simulink model "Md57TrgtPosChk"  (R2018b)
settings: Solver=FixedStepDiscrete  StartTime=0.0  StopTime=10.0  RelTol=1e-3
undefined symbols (not defined in the file or in its folder): Md57TrgtPos_Set, SecRwLtStBkReclnTrgtPos, SecRwLtStFwdBkwdTrgtPos, SecRwLtStLgrstInwdOtwdTrgtPos, SecRwLtStLgrstUpwdDnwdTrgtPos, SecRwLtStZeroTrgtPos
settings Model: Creator=sn2xws  LastModifiedBy=sn2xws
settings Model: ModifiedHistory=|
  | 2024.10.15 V3.0.0 Md57目标位置计算
  | 2024.11.27 V3.0.1 6s版本不看三左前后位置,无解时，使用最小智享位置
settings DataIOCC: SaveFormat=StructureWithTime
settings OptimizationCC: DefaultParameterBehavior=Inlined  EnhancedBackFolding=on  PassReuseOutputArgsAs=Individual arguments  ZeroExternalMemoryAtStartup=off  ZeroInternalMemoryAtStartup=off  OptimizeBlockOrder=speed  DifferentSizesBufferReuse=on  OptimizationCustomize=off
settings DebuggingCC: ParameterTunabilityLossMsg=error
settings SFSimCC: MATLABDynamicMemAlloc=off
settings SFSimCC: SimCustomHeaderCode=|
  | #include "qmath.h"
  | #include "MsminterfDet.h"
  | #include "wisenjoy.h"
settings SFSimCC: SimUserSources=|
  | qmath.c
  | MsminterfDet.c
  | wisenjoy.c
settings RTWCC: SystemTargetFile=autosar.tlc  GenCodeOnly=on  TemplateMakefile=ert_default_tmf  Description=AUTOSAR  GenerateReport=on  IncludeHyperlinkInReport=on  LaunchReport=on  GenerateTraceInfo=on  GenerateTraceReport=on  GenerateTraceReportSl=on  GenerateTraceReportSf=on  GenerateTraceReportEml=on
settings CodeAppCC: ForceParamTrailComments=on  IgnoreCustomStorageClasses=off  OperatorAnnotations=on  SimulinkDataObjDesc=on  SFDataObjDesc=on  InsertBlockDesc=on
settings STFCustomTargetCC: TargetLangStandard=C99 (ISO)  MultiwordLength=256  ParMdlRefBuildCompliant=on  CompOptLevelCompliant=on  IncludeMdlTerminateFcn=off  CombineOutputUpdateFcns=on  SuppressErrorStatus=on  ERTCustomFileBanners=on  SupportNonFinite=off  SupportComplex=off  SupportContinuousTime=off  SupportNonInlinedSFcns=off  RemoveResetFunc=on  MATLABClassNameForMDSCustomization=Simulink.SoftwareTarget.ERTCustomization  AutosarCompliant=on  UseToolchainInfoCompliant=on  LookupTableObjectStructAxisOrder=2,1,3,4,...  LUTObjectStructOrderEvenSpacing=Size,Table,Breakpoints  SystemTargetFile=autosar.tlc
settings ERTTargetCC: TargetLangStandard=C99 (ISO)  ConcurrentExecutionCompliant=off  IncludeMdlTerminateFcn=off  SuppressErrorStatus=on  SupportNonFinite=off  SupportComplex=off  ModelStepFunctionPrototypeControlCompliant=off  CPPClassGenCompliant=off  AutosarCompliant=on  LookupTableObjectStructAxisOrder=2,1,3,4,...  LUTObjectStructOrderEvenSpacing=Size,Table,Breakpoints  InlinedParameterPlacement=NonHierarchical  ERTCustomFileTemplate=example_file_process.tlc  ERTFilePackagingFormat=Compact

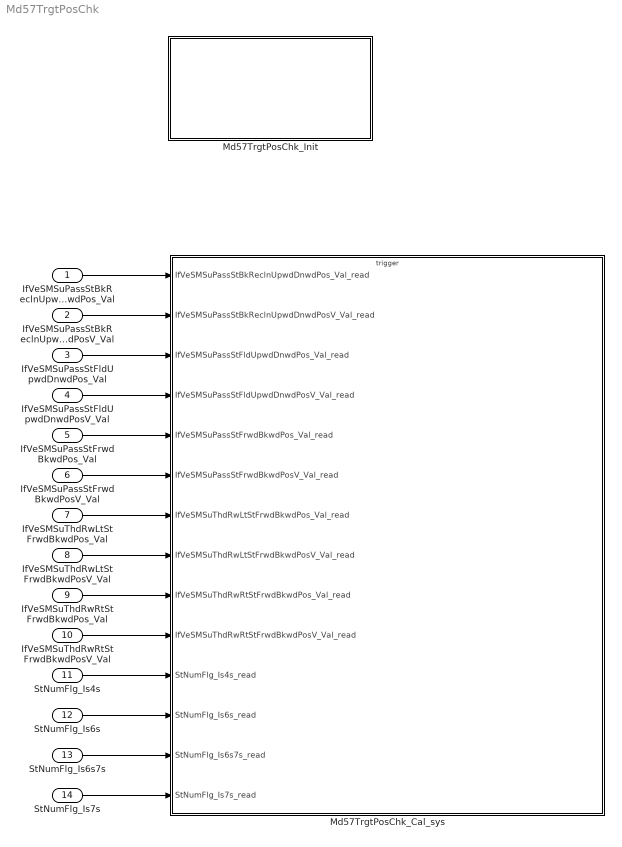
== system Md57TrgtPosChk ==
  IfVeSMSuPassStBkReclnUpwdDnwdPos_Val : Inport  OutDataTypeStr=uint16  PortDimensions=1
  IfVeSMSuPassStBkReclnUpwdDnwdPosV_Val : Inport  Port=2  OutDataTypeStr=boolean  PortDimensions=1
  IfVeSMSuPassStFldUpwdDnwdPos_Val : Inport  Port=3  OutDataTypeStr=uint16  PortDimensions=1
  IfVeSMSuPassStFldUpwdDnwdPosV_Val : Inport  Port=4  OutDataTypeStr=boolean  PortDimensions=1
  IfVeSMSuPassStFrwdBkwdPos_Val : Inport  Port=5  OutDataTypeStr=uint16  PortDimensions=1
  IfVeSMSuPassStFrwdBkwdPosV_Val : Inport  Port=6  OutDataTypeStr=boolean  PortDimensions=1
  IfVeSMSuThdRwLtStFrwdBkwdPos_Val : Inport  Port=7  OutDataTypeStr=uint16  PortDimensions=1
  IfVeSMSuThdRwLtStFrwdBkwdPosV_Val : Inport  Port=8  OutDataTypeStr=boolean  PortDimensions=1
  IfVeSMSuThdRwRtStFrwdBkwdPos_Val : Inport  Port=9  OutDataTypeStr=uint16  PortDimensions=1
  IfVeSMSuThdRwRtStFrwdBkwdPosV_Val : Inport  Port=10  OutDataTypeStr=boolean  PortDimensions=1
  StNumFlg_Is4s : Inport  Port=11  OutDataTypeStr=boolean  PortDimensions=1
  StNumFlg_Is6s : Inport  Port=12  OutDataTypeStr=boolean  PortDimensions=1
  StNumFlg_Is6s7s : Inport  Port=13  OutDataTypeStr=boolean  PortDimensions=1
  StNumFlg_Is7s : Inport  Port=14  OutDataTypeStr=boolean  PortDimensions=1
  Md57TrgtPosChk_Cal_sys : Subsystem
  Md57TrgtPosChk_Init : Subsystem
  wires:
  IfVeSMSuPassStBkReclnUpwdDnwdPos_Val/1 -> Md57TrgtPosChk_Cal_sys/1(IfVeSMSuPassStBkReclnUpwdDnwdPos_Val_read)
  IfVeSMSuPassStBkReclnUpwdDnwdPosV_Val/1 -> Md57TrgtPosChk_Cal_sys/2(IfVeSMSuPassStBkReclnUpwdDnwdPosV_Val_read)
  IfVeSMSuPassStFldUpwdDnwdPos_Val/1 -> Md57TrgtPosChk_Cal_sys/3(IfVeSMSuPassStFldUpwdDnwdPos_Val_read)
  IfVeSMSuPassStFldUpwdDnwdPosV_Val/1 -> Md57TrgtPosChk_Cal_sys/4(IfVeSMSuPassStFldUpwdDnwdPosV_Val_read)
  IfVeSMSuPassStFrwdBkwdPos_Val/1 -> Md57TrgtPosChk_Cal_sys/5(IfVeSMSuPassStFrwdBkwdPos_Val_read)
  IfVeSMSuPassStFrwdBkwdPosV_Val/1 -> Md57TrgtPosChk_Cal_sys/6(IfVeSMSuPassStFrwdBkwdPosV_Val_read)
  IfVeSMSuThdRwLtStFrwdBkwdPos_Val/1 -> Md57TrgtPosChk_Cal_sys/7(IfVeSMSuThdRwLtStFrwdBkwdPos_Val_read)
  IfVeSMSuThdRwLtStFrwdBkwdPosV_Val/1 -> Md57TrgtPosChk_Cal_sys/8(IfVeSMSuThdRwLtStFrwdBkwdPosV_Val_read)
  IfVeSMSuThdRwRtStFrwdBkwdPos_Val/1 -> Md57TrgtPosChk_Cal_sys/9(IfVeSMSuThdRwRtStFrwdBkwdPos_Val_read)
  IfVeSMSuThdRwRtStFrwdBkwdPosV_Val/1 -> Md57TrgtPosChk_Cal_sys/10(IfVeSMSuThdRwRtStFrwdBkwdPosV_Val_read)
  StNumFlg_Is4s/1 -> Md57TrgtPosChk_Cal_sys/11(StNumFlg_Is4s_read)
  StNumFlg_Is6s/1 -> Md57TrgtPosChk_Cal_sys/12(StNumFlg_Is6s_read)
  StNumFlg_Is6s7s/1 -> Md57TrgtPosChk_Cal_sys/13(StNumFlg_Is6s7s_read)
  StNumFlg_Is7s/1 -> Md57TrgtPosChk_Cal_sys/14(StNumFlg_Is7s_read)

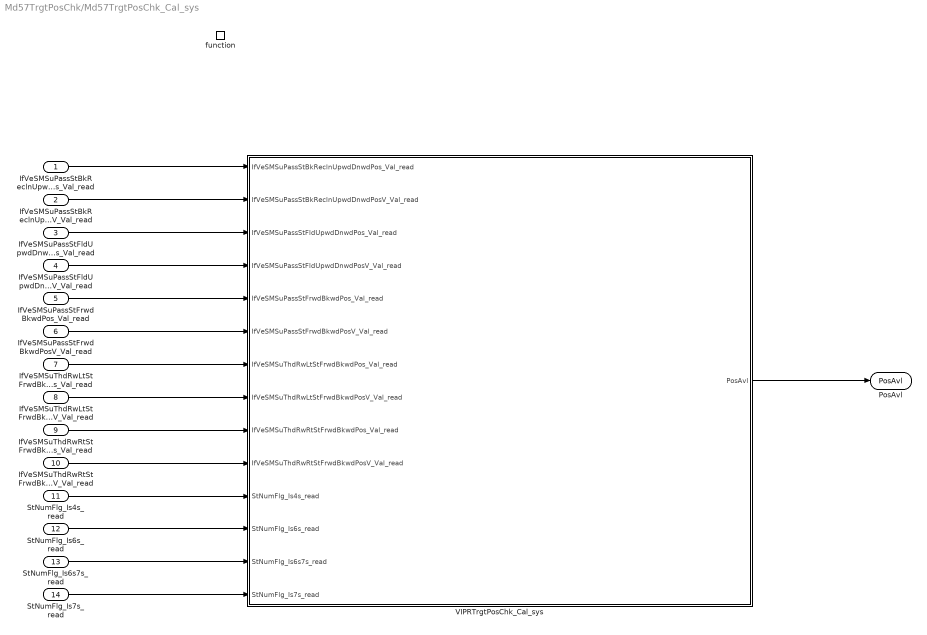
== system Md57TrgtPosChk/Md57TrgtPosChk_Cal_sys ==
  IfVeSMSuPassStBkReclnUpwdDnwdPos_Val_read : Inport
  IfVeSMSuPassStBkReclnUpwdDnwdPosV_Val_read : Inport  Port=2
  IfVeSMSuPassStFldUpwdDnwdPos_Val_read : Inport  Port=3
  IfVeSMSuPassStFldUpwdDnwdPosV_Val_read : Inport  Port=4
  IfVeSMSuPassStFrwdBkwdPos_Val_read : Inport  Port=5
  IfVeSMSuPassStFrwdBkwdPosV_Val_read : Inport  Port=6
  IfVeSMSuThdRwLtStFrwdBkwdPos_Val_read : Inport  Port=7
  IfVeSMSuThdRwLtStFrwdBkwdPosV_Val_read : Inport  Port=8
  IfVeSMSuThdRwRtStFrwdBkwdPos_Val_read : Inport  Port=9
  IfVeSMSuThdRwRtStFrwdBkwdPosV_Val_read : Inport  Port=10
  StNumFlg_Is4s_read : Inport  Port=11
  StNumFlg_Is6s_read : Inport  Port=12
  StNumFlg_Is6s7s_read : Inport  Port=13
  StNumFlg_Is7s_read : Inport  Port=14
  function : TriggerPort  TriggerType=function-call  IsSimulinkFunction=on  FunctionName=Md57TrgtPosChk_Cal  VariantControl=(inherit)
  VIPRTrgtPosChk_Cal_sys : Subsystem
  PosAvl : ArgOut  OutDataTypeStr=uint8  ArgumentName=PosAvl
  wires:
  IfVeSMSuPassStBkReclnUpwdDnwdPos_Val_read/1 -> VIPRTrgtPosChk_Cal_sys/1(IfVeSMSuPassStBkReclnUpwdDnwdPos_Val_read)
  IfVeSMSuPassStBkReclnUpwdDnwdPosV_Val_read/1 -> VIPRTrgtPosChk_Cal_sys/2(IfVeSMSuPassStBkReclnUpwdDnwdPosV_Val_read)
  IfVeSMSuPassStFldUpwdDnwdPos_Val_read/1 -> VIPRTrgtPosChk_Cal_sys/3(IfVeSMSuPassStFldUpwdDnwdPos_Val_read)
  IfVeSMSuPassStFldUpwdDnwdPosV_Val_read/1 -> VIPRTrgtPosChk_Cal_sys/4(IfVeSMSuPassStFldUpwdDnwdPosV_Val_read)
  IfVeSMSuPassStFrwdBkwdPos_Val_read/1 -> VIPRTrgtPosChk_Cal_sys/5(IfVeSMSuPassStFrwdBkwdPos_Val_read)
  IfVeSMSuPassStFrwdBkwdPosV_Val_read/1 -> VIPRTrgtPosChk_Cal_sys/6(IfVeSMSuPassStFrwdBkwdPosV_Val_read)
  IfVeSMSuThdRwLtStFrwdBkwdPos_Val_read/1 -> VIPRTrgtPosChk_Cal_sys/7(IfVeSMSuThdRwLtStFrwdBkwdPos_Val_read)
  IfVeSMSuThdRwLtStFrwdBkwdPosV_Val_read/1 -> VIPRTrgtPosChk_Cal_sys/8(IfVeSMSuThdRwLtStFrwdBkwdPosV_Val_read)
  IfVeSMSuThdRwRtStFrwdBkwdPos_Val_read/1 -> VIPRTrgtPosChk_Cal_sys/9(IfVeSMSuThdRwRtStFrwdBkwdPos_Val_read)
  IfVeSMSuThdRwRtStFrwdBkwdPosV_Val_read/1 -> VIPRTrgtPosChk_Cal_sys/10(IfVeSMSuThdRwRtStFrwdBkwdPosV_Val_read)
  StNumFlg_Is4s_read/1 -> VIPRTrgtPosChk_Cal_sys/11(StNumFlg_Is4s_read)
  StNumFlg_Is6s_read/1 -> VIPRTrgtPosChk_Cal_sys/12(StNumFlg_Is6s_read)
  StNumFlg_Is6s7s_read/1 -> VIPRTrgtPosChk_Cal_sys/13(StNumFlg_Is6s7s_read)
  StNumFlg_Is7s_read/1 -> VIPRTrgtPosChk_Cal_sys/14(StNumFlg_Is7s_read)
  VIPRTrgtPosChk_Cal_sys/1(PosAvl) -> PosAvl/1

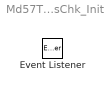
== system Md57TrgtPosChk/Md57TrgtPosChk_Init ==
  Event Listener : EventListener  EventName=reset

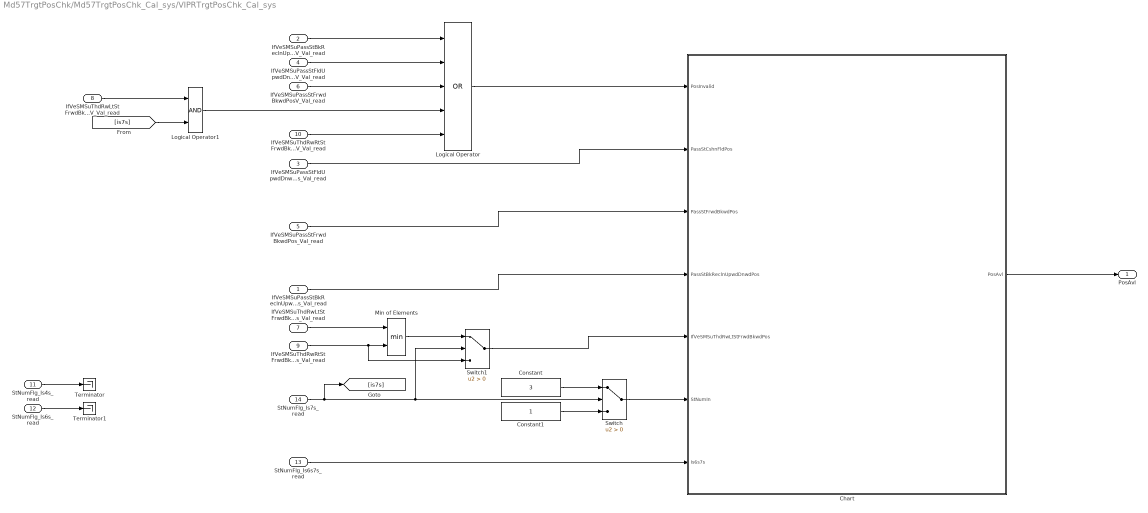
== system Md57TrgtPosChk/Md57TrgtPosChk_Cal_sys/VIPRTrgtPosChk_Cal_sys ==
  IfVeSMSuPassStBkReclnUpwdDnwdPos_Val_read : Inport
  IfVeSMSuPassStBkReclnUpwdDnwdPosV_Val_read : Inport  Port=2
  IfVeSMSuPassStFldUpwdDnwdPos_Val_read : Inport  Port=3
  IfVeSMSuPassStFldUpwdDnwdPosV_Val_read : Inport  Port=4
  IfVeSMSuPassStFrwdBkwdPos_Val_read : Inport  Port=5
  IfVeSMSuPassStFrwdBkwdPosV_Val_read : Inport  Port=6
  IfVeSMSuThdRwLtStFrwdBkwdPos_Val_read : Inport  Port=7
  IfVeSMSuThdRwLtStFrwdBkwdPosV_Val_read : Inport  Port=8
  IfVeSMSuThdRwRtStFrwdBkwdPos_Val_read : Inport  Port=9
  IfVeSMSuThdRwRtStFrwdBkwdPosV_Val_read : Inport  Port=10
  StNumFlg_Is4s_read : Inport  Port=11
  StNumFlg_Is6s_read : Inport  Port=12
  StNumFlg_Is6s7s_read : Inport  Port=13
  StNumFlg_Is7s_read : Inport  Port=14
  Chart : Stateflow chart  TreatAsAtomicUnit=on
  Constant : Constant  Value=3  OutDataTypeStr=uint8
  Constant1 : Constant  OutDataTypeStr=uint8
  Logical Operator : Logic  Operator=OR  Inputs=5  AllPortsSameDT=off  OutDataTypeStr=boolean
  Logical Operator1 : Logic  AllPortsSameDT=off  OutDataTypeStr=boolean
  Min of Elements : MinMax  Inputs=2
  Switch : Switch  Criteria=u2 > Threshold
  Switch1 : Switch  Criteria=u2 > Threshold
  Terminator : Terminator
  Terminator1 : Terminator
  PosAvl : Outport
  wires:
  Chart/1(PosAvl) -> PosAvl/1
  StNumFlg_Is6s7s_read/1 -> Chart/7(Is6s7s)
  StNumFlg_Is4s_read/1 -> Terminator/1
  StNumFlg_Is6s_read/1 -> Terminator1/1
  IfVeSMSuThdRwLtStFrwdBkwdPos_Val_read/1 -> Min of Elements/1
  IfVeSMSuPassStFldUpwdDnwdPosV_Val_read/1 -> Logical Operator/2
  IfVeSMSuPassStBkReclnUpwdDnwdPosV_Val_read/1 -> Logical Operator/1
  IfVeSMSuPassStFrwdBkwdPosV_Val_read/1 -> Logical Operator/3
  IfVeSMSuPassStFrwdBkwdPos_Val_read/1 -> Chart/3(PassStFrwdBkwdPos)
  IfVeSMSuThdRwRtStFrwdBkwdPos_Val_read/1 -> Switch1/3, Min of Elements/2
  IfVeSMSuPassStBkReclnUpwdDnwdPos_Val_read/1 -> Chart/4(PassStBkReclnUpwdDnwdPos)
  IfVeSMSuThdRwRtStFrwdBkwdPosV_Val_read/1 -> Logical Operator/5
  IfVeSMSuPassStFldUpwdDnwdPos_Val_read/1 -> Chart/2(PassStCshnFldPos)
  Logical Operator/1 -> Chart/1(PosInvalid)
  StNumFlg_Is7s_read/1 -> [is7s], Switch1/2, Switch/2
  Constant/1 -> Switch/1
  Constant1/1 -> Switch/3
  Switch/1 -> Chart/6(StNumIn)
  Min of Elements/1 -> Switch1/1
  Switch1/1 -> Chart/5(IfVeSMSuThdRwLtStFrwdBkwdPos)
  [is7s] -> Logical Operator1/2
  IfVeSMSuThdRwLtStFrwdBkwdPosV_Val_read/1 -> Logical Operator1/1
  Logical Operator1/1 -> Logical Operator/4

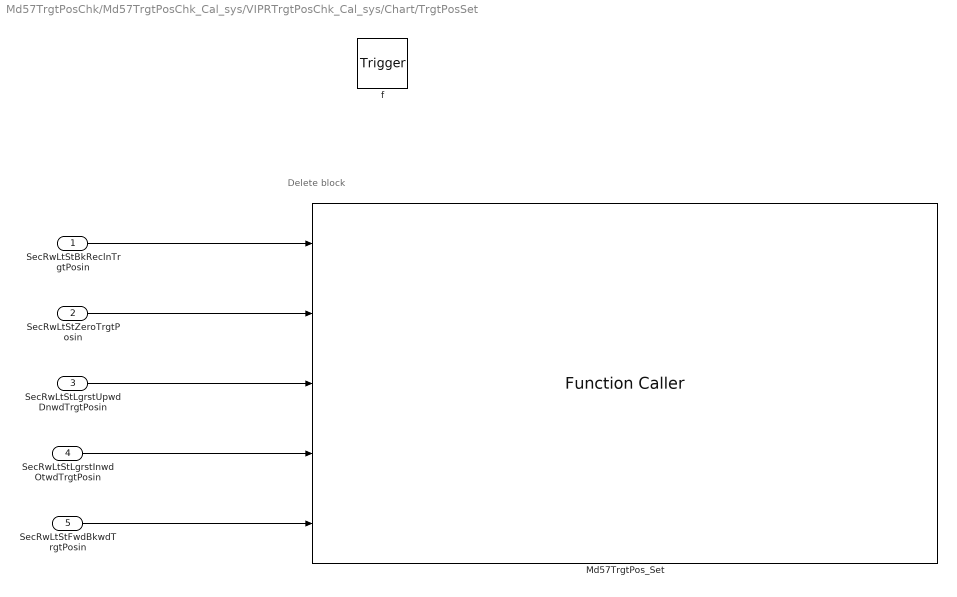
== system Md57TrgtPosChk/Md57TrgtPosChk_Cal_sys/VIPRTrgtPosChk_Cal_sys/Chart/TrgtPosSet ==
  note: Delete block
  SecRwLtStBkReclnTrgtPosin : Inport
  SecRwLtStZeroTrgtPosin : Inport  Port=2
  SecRwLtStLgrstUpwdDnwdTrgtPosin : Inport  Port=3
  SecRwLtStLgrstInwdOtwdTrgtPosin : Inport  Port=4
  SecRwLtStFwdBkwdTrgtPosin : Inport  Port=5
  f : TriggerPort  TriggerType=function-call  VariantControl=(inherit)
      settings: CopyFcn=Stateflow.SLINSF.SimulinkMan.removeBlockPreDeleteFcn  PreDeleteFcn=Stateflow.SLINSF.SimulinkMan.unsafePredeleteFcn
  Md57TrgtPos_Set : FunctionCaller  FunctionPrototype=Md57TrgtPos_Set(SecRwLtStBkReclnTrgtPos,SecRwLtStZeroTrgtPos,SecRwLtStLgrstUpwdDnwdTrgtPos,SecRwLtStLgrstInwdOtwdTrgtPos,SecRwLtStFwdBkwdTrgtPos)  InputArgumentSpecifications=uint16(1), uint16(1), uint16(1), uint16(1), uint16(1)
  wires:
  SecRwLtStBkReclnTrgtPosin/1 -> Md57TrgtPos_Set/1
  SecRwLtStZeroTrgtPosin/1 -> Md57TrgtPos_Set/2
  SecRwLtStLgrstUpwdDnwdTrgtPosin/1 -> Md57TrgtPos_Set/3
  SecRwLtStLgrstInwdOtwdTrgtPosin/1 -> Md57TrgtPos_Set/4
  SecRwLtStFwdBkwdTrgtPosin/1 -> Md57TrgtPos_Set/5

== stateflow chart Md57TrgtPosChk/Md57TrgtPosChk_Cal_sys/VIPRTrgtPosChk_Cal_sys/Chart ==
  state TrgtPosSet(SecRwLtStBkReclnTrgtPosin,SecRwLtStZeroTrgtPosin,SecRwLtStLgrstUpwdDnwdTrgtPosin,SecRwLtStLgrstInwdOtwdTrgtPosin,SecRwLtStFwdBkwdTrgtPosin) [function]
  (default) -> (junction 2)
  (junction 2) -> (junction 6) [order 1] : [PosInvalid||!Is6s7s]
  (junction 2) -> (junction 172) [order 2]
  (junction 6) -> (junction 158)
  (junction 172) -> (junction 174) [order 1] : [PassStCshnFldPos==0]
  (junction 172) -> (junction 178) [order 2] : {
      | r1mhin= 0.4188;
      | r1mbin = PassStBkReclnUpwdDnwdPos;
      | r1mbin = r1mbin/4000;
      | }
  (junction 174) -> (junction 176) : {
      | r1mhin = 1;
      | r1mbin = 0;
      | }
  (junction 176) -> (junction 178)
  (junction 178) -> (junction 53) : {
      | r1mfin = PassStFrwdBkwdPos;
      | r1mfin = r1mfin/4000;
      | r3mfin = IfVeSMSuThdRwLtStFrwdBkwdPos;
      | r3mfin = r3mfin/4000;
      | }
  (junction 53) -> (junction 158) [order 1] : [MsmInterfDet_WisdomEnjoySearch(StNumIn,r1mhin,r1mbin,r1mfin,r3mfin)<=0]
  (junction 53) -> (junction 100) [order 2] : {
      | ans = MsmInterfDet_GetAns();
      | }
  (junction 158) -> (junction 8) : {PosAvl = 1;
      | TrgtPosSet(1902,0,2400,4000,4000);}
  (junction 100) -> (junction 4) : {
      | SecRwLtFwdBkwdTrgtPos = ans.ans_r2mf*4000;
      | SecRwLtStZeroTrgtPos = ans.ans_r2m0*4000;
      | SecRwLtStBkReclnTrgtPos =ans.ans_r2mb*4000;
      | SecRwLtStLgrstUpwdDnwdTrgtPos = ans.ans_r2ml*4000;
      | %SecRwLtStLgrstInwdOtwdTrgtPos =ans.ans_r2me*4000;
      | SecRwLtStLgrstInwdOtwdTrgtPos = 4000;
      | TrgtPosSet(SecRwLtStBkReclnTrgtPos,SecRwLtStZeroTrgtPos,SecRwLtStLgrstUpwdDnwdTrgtPos,SecRwLtStLgrstInwdOtwdTrgtPos,SecRwLtFwdBkwdTrgtPos);
      | PosAvl = 1;
      | }
  (junction 8) -> (junction 4)
  (junction 4) -> (junction 96)
  data: SecRwLtStBkReclnTrgtPosin function_input; SecRwLtStZeroTrgtPosin function_input; SecRwLtStLgrstUpwdDnwdTrgtPosin function_input; SecRwLtStLgrstInwdOtwdTrgtPosin function_input; SecRwLtStFwdBkwdTrgtPosin function_input; PosAvl output; SecRwLtStBkReclnTrgtPos local uint16; SecRwLtStZeroTrgtPos local uint16; SecRwLtStLgrstUpwdDnwdTrgtPos local uint16; SecRwLtStLgrstInwdOtwdTrgtPos local uint16; SecRwLtFwdBkwdTrgtPos local uint16; PosInvalid input boolean; PassStCshnFldPos input uint16; PassStFrwdBkwdPos input uint16; PassStBkReclnUpwdDnwdPos input uint16; IfVeSMSuThdRwLtStFrwdBkwdPos input uint16; r1mhin local single; r1mbin local single; r1mfin local single; r3mfin local single; ans local Bus: MsmAnsTyp; StNumIn input uint8; Is6s7s input boolean
